simulink library "Project3_lib"  (R2017b)
settings: Solver=ode45  StartTime=0.0  StopTime=10.0  RelTol=1e-3
values from neighbouring files (symbols this model uses):
  C = 1e-3    (= 0.001)    [init.m]    (also in prob1_Torque_vs_speed.m; prob2.m)
  Kd = 0.5    [init.m]
  Kq = 0.5    [init.m]
  L = 5e-6    (= 5e-06)    [init.m]    (also in prob1_Torque_vs_speed.m; prob2.m)
  lambda_m = 0.1062    [init.m]    (also in prob2.m)
  Ld = 0.3e-3    (= 0.0003)    [init.m]    (also in prob1_Torque_vs_speed.m; prob2.m)
  Lq = 0.3e-3    (= 0.0003)    [init.m]    (also in prob1_Torque_vs_speed.m; prob2.m)
  P = 6    [init.m]    (also in prob1_Torque_vs_speed.m; prob2.m)
  R = 0.01    [init.m]    (also in prob1_Torque_vs_speed.m; prob2.m)
  rs = 0.01    [init.m]    (also in prob1_Torque_vs_speed.m; prob2.m)
  V_batt = 350    [init.m]    (also in prob1_Torque_vs_speed.m; prob2.m)
libraries: simulink x1
settings Model: Creator=wasynczu  LastModifiedBy=khan1
settings DataIOCC: SaveFormat=StructureWithTime
settings OptimizationCC: LifeSpan=inf
settings DebuggingCC: SFExecutionAtInitializationDiag=none
settings HardwareCC: ProdBitPerSizeT=32  ProdBitPerPtrDiffT=32  ProdWordSize=32  ProdHWDeviceType=Specified
settings SFSimCC: SimUseLocalCustomCode=on
settings RTWCC: RTWUseLocalCustomCode=on
settings CodeAppCC: StateflowObjectComments=on

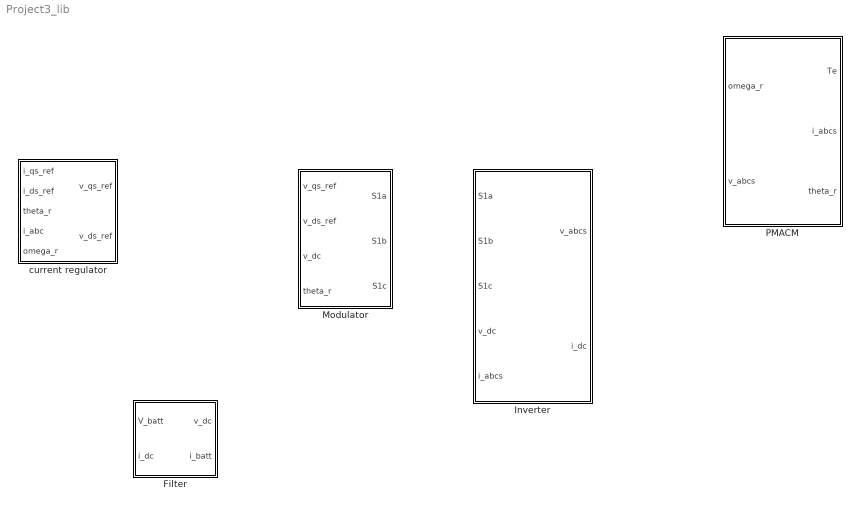
== system Project3_lib ==
  Filter : Subsystem
  Inverter : Subsystem
  Modulator : Subsystem
  PMACM : Subsystem
  current regulator : Subsystem

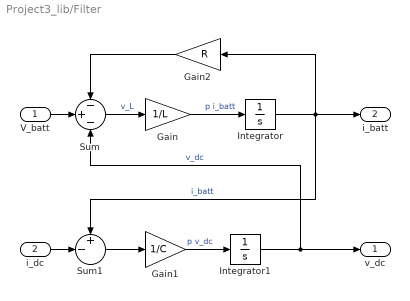
== system Project3_lib/Filter ==
  V_batt : Inport
  i_dc : Inport  Port=2
  Gain : Gain  Gain=1/L
  Gain1 : Gain  Gain=1/C
  Gain2 : Gain  Gain=R
  Integrator : Integrator
  Integrator1 : Integrator  InitialCondition=V_batt
  Sum : Sum  Inputs=-+-
  Sum1 : Sum  Inputs=+-|
  v_dc : Outport
  i_batt : Outport  Port=2
  wires:
  Sum/1 -> Gain/1  "v_L"
  Gain/1 -> Integrator/1  "p i_batt"
  Integrator/1 -> Gain2/1, i_batt/1, Sum1/1  "i_batt"
  i_dc/1 -> Sum1/2
  Sum1/1 -> Gain1/1
  Integrator1/1 -> v_dc/1, Sum/3  "v_dc"
  V_batt/1 -> Sum/2
  Gain2/1 -> Sum/1
  Gain1/1 -> Integrator1/1  "p v_dc"

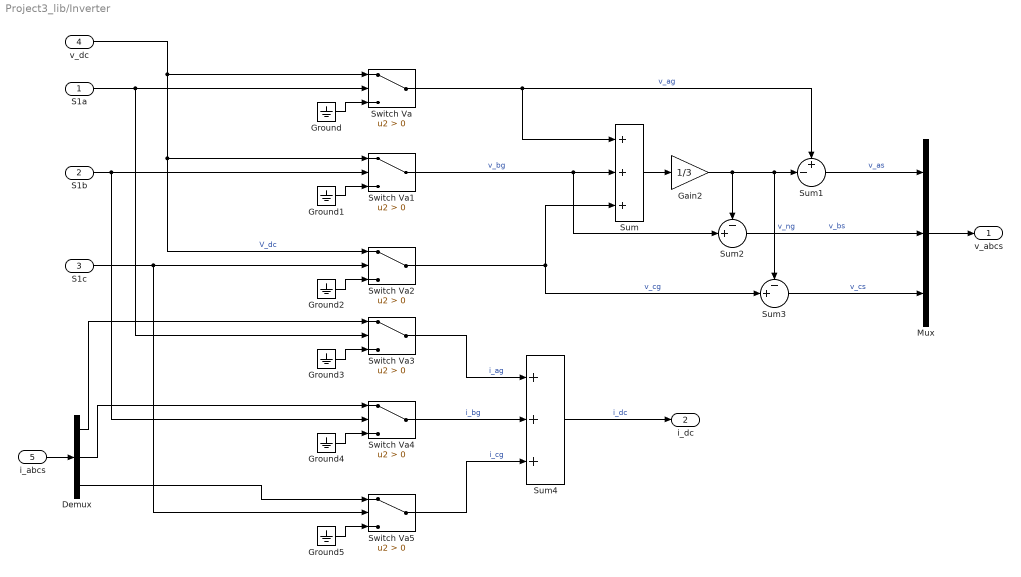
== system Project3_lib/Inverter ==
  S1a : Inport
  S1b : Inport  Port=2
  S1c : Inport  Port=3
  v_dc : Inport  Port=4
  i_abcs : Inport  Port=5
  Demux : Demux  Outputs=3
  Gain2 : Gain  Gain=1/3
  Ground{,1..5} (6 alike) : Ground
  Mux : Mux  Inputs=3
  Sum : Sum  Inputs=+++
  Sum1 : Sum  Inputs=+-|
  Sum2 : Sum  Inputs=-+|
  Sum3 : Sum  Inputs=-+|
  Sum4 : Sum  Inputs=+++
  Switch Va{,1..5} (6 alike) : Switch  Criteria=u2 > Threshold
  v_abcs : Outport
  i_dc : Outport  Port=2
  wires:
  Ground/1 -> Switch Va/3
  Ground1/1 -> Switch Va1/3
  Ground2/1 -> Switch Va2/3
  v_dc/1 -> Switch Va1/1, Switch Va2/1, Switch Va/1  "V_dc"
  S1a/1 -> Switch Va/2, Switch Va3/2
  S1b/1 -> Switch Va1/2, Switch Va4/2
  S1c/1 -> Switch Va2/2, Switch Va5/2
  Switch Va/1 -> Sum/1, Sum1/1  "v_ag"
  Switch Va1/1 -> Sum/2, Sum2/2  "v_bg"
  Switch Va2/1 -> Sum/3, Sum3/2  "v_cg"
  Sum/1 -> Gain2/1
  Gain2/1 -> Sum2/1, Sum1/2, Sum3/1  "v_ng"
  Ground3/1 -> Switch Va3/3
  Ground4/1 -> Switch Va4/3
  Ground5/1 -> Switch Va5/3
  Switch Va3/1 -> Sum4/1  "i_ag"
  Switch Va4/1 -> Sum4/2  "i_bg"
  Switch Va5/1 -> Sum4/3  "i_cg"
  Sum2/1 -> Mux/2  "v_bs"
  Sum3/1 -> Mux/3  "v_cs"
  Demux/2 -> Switch Va4/1
  Sum4/1 -> i_dc/1  "i_dc"
  Demux/3 -> Switch Va5/1
  i_abcs/1 -> Demux/1
  Demux/1 -> Switch Va3/1
  Mux/1 -> v_abcs/1
  Sum1/1 -> Mux/1  "v_as"

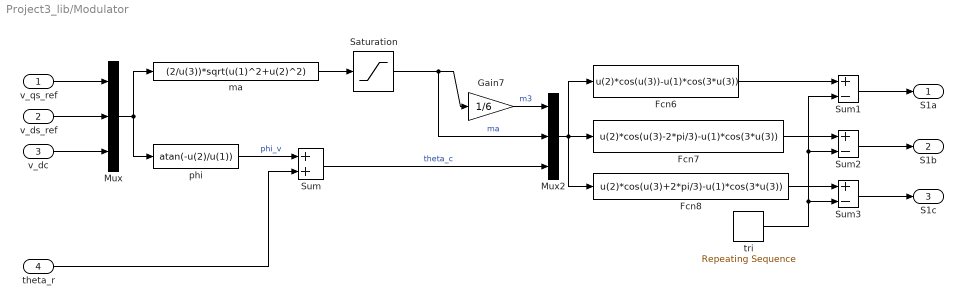
== system Project3_lib/Modulator ==
  v_qs_ref : Inport
  v_ds_ref : Inport  Port=2
  v_dc : Inport  Port=3
  theta_r : Inport  Port=4
  Fcn6 : Fcn  Expr=u(2)*cos(u(3))-u(1)*cos(3*u(3))
  Fcn7 : Fcn  Expr=u(2)*cos(u(3)-2*pi/3)-u(1)*cos(3*u(3))
  Fcn8 : Fcn  Expr=u(2)*cos(u(3)+2*pi/3)-u(1)*cos(3*u(3))
  Gain7 : Gain  Gain=1/6
  Mux : Mux  Inputs=3
  Mux2 : Mux  Inputs=3
  Saturation : Saturate  UpperLimit=2/sqrt(3)  LowerLimit=0
  Sum : Sum
  Sum1 : Sum  Inputs=+-
  Sum2 : Sum  Inputs=+-
  Sum3 : Sum  Inputs=+-
  ma : Fcn  Expr=(2/u(3))*sqrt(u(1)^2+u(2)^2)
  phi : Fcn  Expr=atan(-u(2)/u(1))
  tri : simulink/Sources/Repeating Sequence  rep_seq_t=[0 1/40000 1/20000 3/40000 1/10000]  rep_seq_y=[0 1 0 -1 0]
  S1a : Outport
  S1b : Outport  Port=2
  S1c : Outport  Port=3
  wires:
  tri/1 -> Sum3/2, Sum2/2, Sum1/2
  Sum1/1 -> S1a/1
  Sum2/1 -> S1b/1
  Sum3/1 -> S1c/1
  v_qs_ref/1 -> Mux/1
  v_ds_ref/1 -> Mux/2
  v_dc/1 -> Mux/3
  Mux/1 -> ma/1, phi/1
  phi/1 -> Sum/1  "phi_v"
  Sum/1 -> Mux2/3  "theta_c"
  Mux2/1 -> Fcn6/1, Fcn7/1, Fcn8/1
  Gain7/1 -> Mux2/1  "m3"
  Fcn6/1 -> Sum1/1
  Fcn7/1 -> Sum2/1
  Fcn8/1 -> Sum3/1
  ma/1 -> Saturation/1
  Saturation/1 -> Gain7/1, Mux2/2  "ma"
  theta_r/1 -> Sum/2

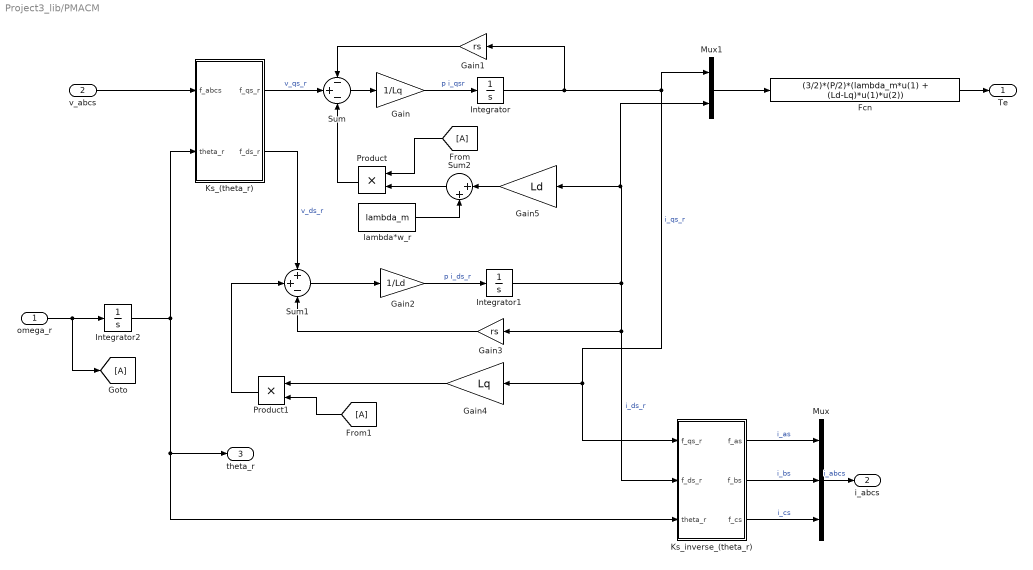
== system Project3_lib/PMACM ==
  omega_r : Inport
  v_abcs : Inport  Port=2
  Fcn : Fcn  Expr=(3/2)*(P/2)*(lambda_m*u(1) + (Ld-Lq)*u(1)*u(2))
  Gain : Gain  Gain=1/Lq
  Gain1 : Gain  Gain=rs
  Gain2 : Gain  Gain=1/Ld
  Gain3 : Gain  Gain=rs
  Gain4 : Gain  Gain=Lq
  Gain5 : Gain  Gain=Ld
  Integrator : Integrator
  Integrator1 : Integrator
  Integrator2 : Integrator
  Ks_(theta_r) : Subsystem
  Ks_inverse_(theta_r) : Subsystem
  Mux : Mux  Inputs=3
  Mux1 : Mux  Inputs=2
  Product : Product
  Product1 : Product
  Sum : Sum  Inputs=-+-
  Sum1 : Sum  Inputs=++-
  Sum2 : Sum  Inputs=|++
  lambda*w_r : Constant  Value=lambda_m
  Te : Outport
  i_abcs : Outport  Port=2
  theta_r : Outport  Port=3
  wires:
  Ks_(theta_r)/2(f_ds_r) -> Sum1/1  "v_ds_r"
  Ks_(theta_r)/1(f_qs_r) -> Sum/2  "v_qs_r"
  Sum/1 -> Gain/1
  Gain/1 -> Integrator/1  "p i_qsr"
  Integrator/1 -> Mux1/1, Gain4/1, Ks_inverse_(theta_r)/1(f_qs_r), Gain1/1  "i_qs_r"
  Sum1/1 -> Gain2/1
  Gain2/1 -> Integrator1/1  "p i_ds_r"
  Integrator1/1 -> Mux1/2, Gain5/1, Gain3/1, Ks_inverse_(theta_r)/2(f_ds_r)  "i_ds_r"
  Gain3/1 -> Sum1/3
  Integrator2/1 -> Ks_(theta_r)/2(theta_r), Ks_inverse_(theta_r)/3(theta_r), theta_r/1
  Ks_inverse_(theta_r)/1(f_as) -> Mux/1  "i_as"
  Ks_inverse_(theta_r)/2(f_bs) -> Mux/2  "i_bs"
  Ks_inverse_(theta_r)/3(f_cs) -> Mux/3  "i_cs"
  Fcn/1 -> Te/1
  Mux/1 -> i_abcs/1  "i_abcs"
  v_abcs/1 -> Ks_(theta_r)/1(f_abcs)
  omega_r/1 -> [A], Integrator2/1
  Gain5/1 -> Sum2/1
  lambda*w_r/1 -> Sum2/2
  Sum2/1 -> Product/2
  Gain1/1 -> Sum/1
  Product/1 -> Sum/3
  [A] -> Product/1
  Gain4/1 -> Product1/1
  Product1/1 -> Sum1/2
  [A] -> Product1/2
  Mux1/1 -> Fcn/1

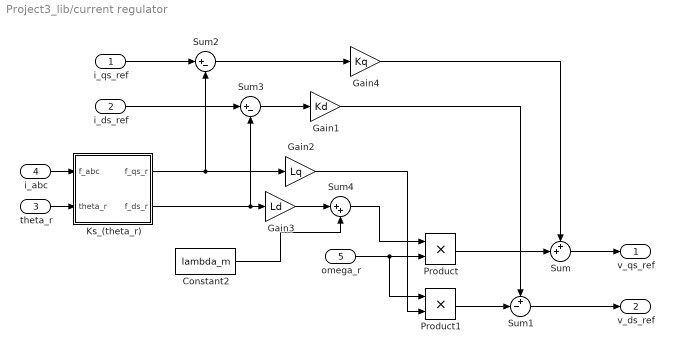
== system Project3_lib/current regulator ==
  i_qs_ref : Inport
  i_ds_ref : Inport  Port=2
  theta_r : Inport  Port=3
  i_abc : Inport  Port=4
  omega_r : Inport  Port=5
  Constant2 : Constant  Value=lambda_m
  Gain1 : Gain  Gain=Kd
  Gain2 : Gain  Gain=Lq
  Gain3 : Gain  Gain=Ld
  Gain4 : Gain  Gain=Kq
  Ks_(theta_r) : Subsystem
  Product : Product
  Product1 : Product
  Sum : Sum  Inputs=++|
  Sum1 : Sum  Inputs=+-|
  Sum2 : Sum  Inputs=|+-
  Sum3 : Sum  Inputs=|+-
  Sum4 : Sum  Inputs=|++
  v_qs_ref : Outport
  v_ds_ref : Outport  Port=2
  wires:
  theta_r/1 -> Ks_(theta_r)/2(theta_r)
  Product/1 -> Sum/2
  omega_r/1 -> Product1/1, Product/2
  Sum/1 -> v_qs_ref/1
  Product1/1 -> Sum1/2
  Sum1/1 -> v_ds_ref/1
  Sum3/1 -> Gain1/1
  Sum2/1 -> Gain4/1
  Gain1/1 -> Sum1/1
  i_ds_ref/1 -> Sum3/1
  i_qs_ref/1 -> Sum2/1
  i_abc/1 -> Ks_(theta_r)/1(f_abc)
  Ks_(theta_r)/1(f_qs_r) -> Gain2/1, Sum2/2
  Ks_(theta_r)/2(f_ds_r) -> Sum3/2, Gain3/1
  Gain2/1 -> Product1/2
  Gain3/1 -> Sum4/1
  Sum4/1 -> Product/1
  Constant2/1 -> Sum4/2
  Gain4/1 -> Sum/1

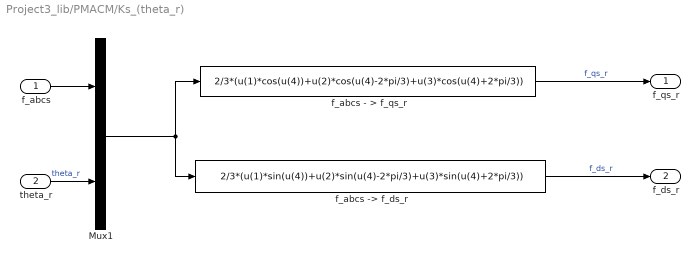
== system Project3_lib/PMACM/Ks_(theta_r) ==
  f_abcs : Inport
  theta_r : Inport  Port=2
  Mux1 : Mux  Inputs=2
  f_abcs - > f_qs_r : Fcn  Expr=2/3*(u(1)*cos(u(4))+u(2)*cos(u(4)-2*pi/3)+u(3)*cos(u(4)+2*pi/3))
  "f_abcs -> f_ds_r" : Fcn  Expr=2/3*(u(1)*sin(u(4))+u(2)*sin(u(4)-2*pi/3)+u(3)*sin(u(4)+2*pi/3))
  f_qs_r : Outport
  f_ds_r : Outport  Port=2
  wires:
  "f_abcs -> f_ds_r"/1 -> f_ds_r/1  "f_ds_r"
  f_abcs/1 -> Mux1/1
  f_abcs - > f_qs_r/1 -> f_qs_r/1  "f_qs_r"
  Mux1/1 -> "f_abcs -> f_ds_r"/1, f_abcs - > f_qs_r/1
  theta_r/1 -> Mux1/2  "theta_r"

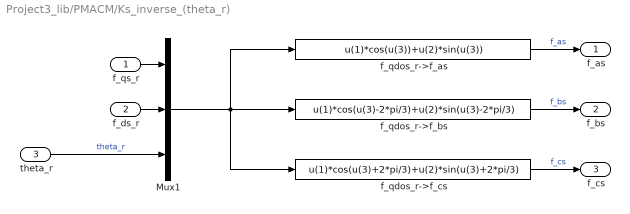
== system Project3_lib/PMACM/Ks_inverse_(theta_r) ==
  f_qs_r : Inport
  f_ds_r : Inport  Port=2
  theta_r : Inport  Port=3
  Mux1 : Mux  Inputs=3
  f_qdos_r->f_as : Fcn  Expr=u(1)*cos(u(3))+u(2)*sin(u(3))
  f_qdos_r->f_bs : Fcn  Expr=u(1)*cos(u(3)-2*pi/3)+u(2)*sin(u(3)-2*pi/3)
  f_qdos_r->f_cs : Fcn  Expr=u(1)*cos(u(3)+2*pi/3)+u(2)*sin(u(3)+2*pi/3)
  f_as : Outport
  f_bs : Outport  Port=2
  f_cs : Outport  Port=3
  wires:
  theta_r/1 -> Mux1/3  "theta_r"
  Mux1/1 -> f_qdos_r->f_as/1, f_qdos_r->f_bs/1, f_qdos_r->f_cs/1
  f_qdos_r->f_as/1 -> f_as/1  "f_as"
  f_qs_r/1 -> Mux1/1
  f_ds_r/1 -> Mux1/2
  f_qdos_r->f_bs/1 -> f_bs/1  "f_bs"
  f_qdos_r->f_cs/1 -> f_cs/1  "f_cs"

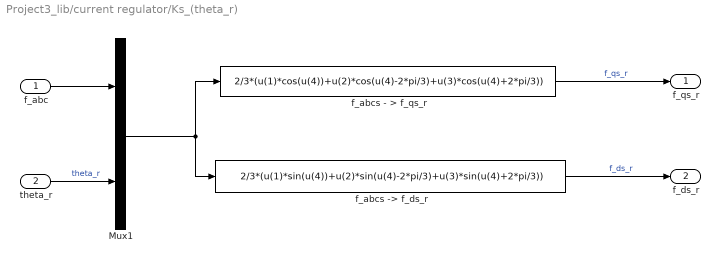
== system Project3_lib/current regulator/Ks_(theta_r) ==
  f_abc : Inport
  theta_r : Inport  Port=2
  Mux1 : Mux  Inputs=2
  f_abcs - > f_qs_r : Fcn  Expr=2/3*(u(1)*cos(u(4))+u(2)*cos(u(4)-2*pi/3)+u(3)*cos(u(4)+2*pi/3))
  "f_abcs -> f_ds_r" : Fcn  Expr=2/3*(u(1)*sin(u(4))+u(2)*sin(u(4)-2*pi/3)+u(3)*sin(u(4)+2*pi/3))
  f_qs_r : Outport
  f_ds_r : Outport  Port=2
  wires:
  "f_abcs -> f_ds_r"/1 -> f_ds_r/1  "f_ds_r"
  f_abc/1 -> Mux1/1
  f_abcs - > f_qs_r/1 -> f_qs_r/1  "f_qs_r"
  Mux1/1 -> "f_abcs -> f_ds_r"/1, f_abcs - > f_qs_r/1
  theta_r/1 -> Mux1/2  "theta_r"
